simulink library "SUB_ECU_L4_MABX_HW_Interface_PTC_166"  (R2018a)
settings: Solver=VariableStepAuto  StartTime=0.0  StopTime=10.0  RelTol=1e-3
PostLoadFcn:
  | , if any(exist('dsrtsu_mdlpostloadfcn', 'file') == [2, 3, 6]), try dsrtsu_mdlpostloadfcn('Execute', bdroot); catch fprintf('Error in PostLoadFcn (dsrtsu_mdlpostloadfcn) for model "%s":\n %s\n', bdroot, lasterr); end, end,
undefined symbols (not defined in the file or in its folder): CANR_PROPB_REAX_3_13_CHANNEL_APV, CANR_PROPB_REAX_4_13_CHANNEL_APV, CANR_PROPB_XPR_1_50_CHANNEL_APV, ENUM_CAN_RX_T, ENUM_CAN_TX_T, ENUM_REAX_OPERATION_MODE_T, ENUM_SIGNAL_HEALTH_T, ENUM_XBR_CONTROL_MODE_T, ENUM_XBR_EBI_MODE_T, ENUM_XBR_PASS_THROUGH_ACTIVE_T, ENUM_XBR_PRIORITY_T, ENUM_XPR_INHIBIT_PARK_MANUAL_T, ENUM_XPR_INHIBIT_UNPARK_MANUAL_T, ENUM_XPR_PARK_MANUAL_T, ENUM_XPR_UNPARK_MANUAL_T, PROPB_REAX_1_E4_DES_POS_SIG_SRC_APV, PROPB_REAX_1_E4_DESIRED_OPMODE_APV, PROPB_REAX_1_E4_DESIRED_POSITION_APV, ptc_matlab_lib
libraries: PTC_MBDS_LIB x163, rtican x79, simulink x41, EmE_MBD_Blockset x35, rti1401lib_dio_type4 x8, simulink_need_slupdate x7, $bdroot x5, rti1401lib_adc_type4 x3, rtitasklib x1
(part 5 of 25)

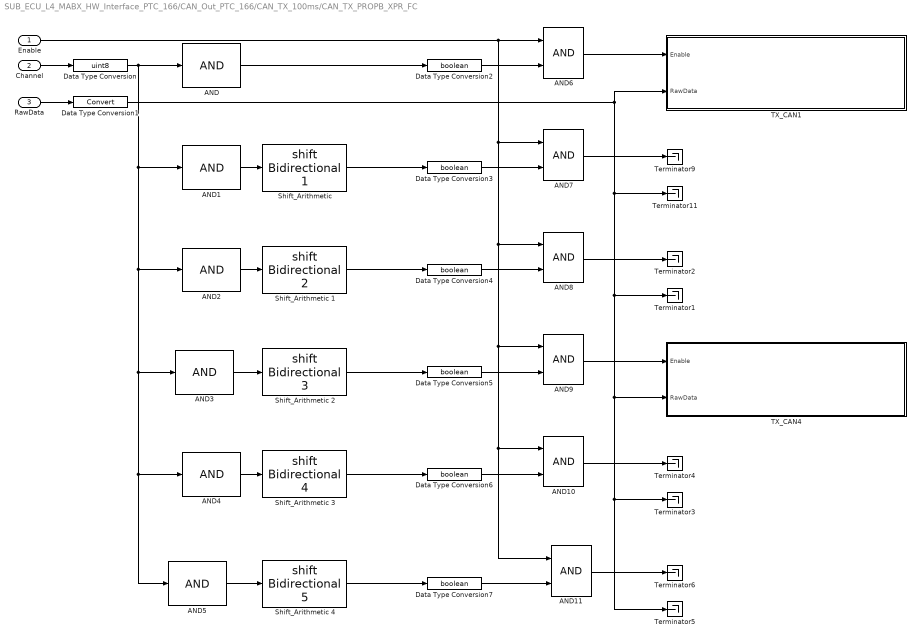
== system SUB_ECU_L4_MABX_HW_Interface_PTC_166/CAN_Out_PTC_166/CAN_TX_100ms/CAN_TX_PROPB_XPR_FC ==
  Enable : Inport
  Channel : Inport  Port=2  OutDataTypeStr=Enum: ENUM_CAN_TX_T
  RawData : Inport  Port=3  OutDataTypeStr=uint8
  AND : PTC_MBDS_LIB/MBDS Standard Library/Basic Operations/Logic and Bit Operations/AND  BitwiseMode=on  Inputs=1  UseBitMask=on  BitMask=bin2dec('00000001')  OutDataTypeStr=Inherit: Inherit via back propagation  PTC_MBDS_BlockVersion=5.41  PTC_BlockType=PTC_MBDS_AND
      settings: AttributesFormatString=bitwise  SourceProductName=PACCAR Technical Center MBDS Library
  AND1 : PTC_MBDS_LIB/MBDS Standard Library/Basic Operations/Logic and Bit Operations/AND  BitwiseMode=on  Inputs=1  UseBitMask=on  BitMask=bin2dec('00000010')  OutDataTypeStr=Inherit: Inherit via back propagation  PTC_MBDS_BlockVersion=5.41  PTC_BlockType=PTC_MBDS_AND
      settings: AttributesFormatString=bitwise  SourceProductName=PACCAR Technical Center MBDS Library
  AND{6..11} (6 alike) : PTC_MBDS_LIB/MBDS Standard Library/Basic Operations/Logic and Bit Operations/AND  BitwiseMode=off  Inputs=2  UseBitMask=off  BitMask='A7'  OutDataTypeStr=Inherit: Inherit via back propagation  PTC_MBDS_BlockVersion=5.41  PTC_BlockType=PTC_MBDS_AND
      settings: SourceProductName=PACCAR Technical Center MBDS Library
  AND2 : PTC_MBDS_LIB/MBDS Standard Library/Basic Operations/Logic and Bit Operations/AND  BitwiseMode=on  Inputs=1  UseBitMask=on  BitMask=bin2dec('00000100')  OutDataTypeStr=Inherit: Inherit via back propagation  PTC_MBDS_BlockVersion=5.41  PTC_BlockType=PTC_MBDS_AND
      settings: AttributesFormatString=bitwise  SourceProductName=PACCAR Technical Center MBDS Library
  AND3 : PTC_MBDS_LIB/MBDS Standard Library/Basic Operations/Logic and Bit Operations/AND  BitwiseMode=on  Inputs=1  UseBitMask=on  BitMask=bin2dec('00001000')  OutDataTypeStr=Inherit: Inherit via back propagation  PTC_MBDS_BlockVersion=5.41  PTC_BlockType=PTC_MBDS_AND
      settings: AttributesFormatString=bitwise  SourceProductName=PACCAR Technical Center MBDS Library
  AND4 : PTC_MBDS_LIB/MBDS Standard Library/Basic Operations/Logic and Bit Operations/AND  BitwiseMode=on  Inputs=1  UseBitMask=on  BitMask=bin2dec('00010000')  OutDataTypeStr=Inherit: Inherit via back propagation  PTC_MBDS_BlockVersion=5.41  PTC_BlockType=PTC_MBDS_AND
      settings: AttributesFormatString=bitwise  SourceProductName=PACCAR Technical Center MBDS Library
  AND5 : PTC_MBDS_LIB/MBDS Standard Library/Basic Operations/Logic and Bit Operations/AND  BitwiseMode=on  Inputs=1  UseBitMask=on  BitMask=bin2dec('00100000')  OutDataTypeStr=Inherit: Inherit via back propagation  PTC_MBDS_BlockVersion=5.41  PTC_BlockType=PTC_MBDS_AND
      settings: AttributesFormatString=bitwise  SourceProductName=PACCAR Technical Center MBDS Library
  Data Type Conversion : DataTypeConversion  OutDataTypeStr=uint8  SaturateOnIntegerOverflow=on
  Data Type Conversion1 : DataTypeConversion  SaturateOnIntegerOverflow=on
  Data Type Conversion{2..7} (6 alike) : DataTypeConversion  OutDataTypeStr=boolean  SaturateOnIntegerOverflow=on
  "Shift_Arithmetic " : ArithShift  BitShiftNumber=1
  Shift_Arithmetic 1 : ArithShift  BitShiftNumber=2
  Shift_Arithmetic 2 : ArithShift  BitShiftNumber=3
  Shift_Arithmetic 3 : ArithShift  BitShiftNumber=4
  Shift_Arithmetic 4 : ArithShift  BitShiftNumber=5
  TX_CAN1 : Subsystem
  TX_CAN4 : Subsystem
  Terminator{1..6,9,11} (8 alike) : Terminator
  wires:
  Shift_Arithmetic 4/1 -> Data Type Conversion7/1
  AND5/1 -> Shift_Arithmetic 4/1
  Shift_Arithmetic 3/1 -> Data Type Conversion6/1
  AND4/1 -> Shift_Arithmetic 3/1
  Shift_Arithmetic 2/1 -> Data Type Conversion5/1
  AND3/1 -> Shift_Arithmetic 2/1
  Shift_Arithmetic 1/1 -> Data Type Conversion4/1
  "Shift_Arithmetic "/1 -> Data Type Conversion3/1
  AND/1 -> Data Type Conversion2/1
  RawData/1 -> Data Type Conversion1/1
  Data Type Conversion/1 -> AND2/1, AND3/1, AND5/1, AND4/1, AND1/1, AND/1
  Channel/1 -> Data Type Conversion/1
  AND2/1 -> Shift_Arithmetic 1/1
  AND1/1 -> "Shift_Arithmetic "/1
  Data Type Conversion1/1 -> TX_CAN1/2(RawData), Terminator11/1, Terminator1/1, TX_CAN4/2(RawData), Terminator5/1, Terminator3/1
  Data Type Conversion2/1 -> AND6/2
  Data Type Conversion3/1 -> AND7/2
  Data Type Conversion4/1 -> AND8/2
  Data Type Conversion5/1 -> AND9/2
  Data Type Conversion6/1 -> AND10/2
  Data Type Conversion7/1 -> AND11/2
  Enable/1 -> AND11/1, AND10/1, AND9/1, AND8/1, AND7/1, AND6/1
  AND11/1 -> Terminator6/1
  AND10/1 -> Terminator4/1
  AND9/1 -> TX_CAN4/1(Enable)
  AND8/1 -> Terminator2/1
  AND7/1 -> Terminator9/1
  AND6/1 -> TX_CAN1/1(Enable)

== system SUB_ECU_L4_MABX_HW_Interface_PTC_166/CAN_Out_PTC_166/CAN_TX_100ms/COGSRapidUpdate ==
  Enable : Inport
  Data : Inport  Port=2
  Data Type Conversion2 : DataTypeConversion  OutDataTypeStr=boolean  SaturateOnIntegerOverflow=on
  TX : Subsystem
  wires:
  Enable/1 -> Data Type Conversion2/1
  Data/1 -> TX/2(Data)
  Data Type Conversion2/1 -> TX/1(Enable)

== system SUB_ECU_L4_MABX_HW_Interface_PTC_166/CAN_Out_PTC_166/CAN_TX_100ms/EBC1_8B ==
  Enable : Inport
  Data : Inport  Port=2
  Data Type Conversion2 : DataTypeConversion  OutDataTypeStr=boolean  SaturateOnIntegerOverflow=on
  TX_EBC1_8B : Subsystem
  wires:
  Data Type Conversion2/1 -> TX_EBC1_8B/1(Enable)
  Data/1 -> TX_EBC1_8B/2(Data)
  Enable/1 -> Data Type Conversion2/1

== system SUB_ECU_L4_MABX_HW_Interface_PTC_166/CAN_Out_PTC_166/CAN_TX_100ms/EffortsValue ==
  Constant : Constant  Value=int16(512)
  EffortsValue : Outport
  wires:
  Constant/1 -> EffortsValue/1

== system SUB_ECU_L4_MABX_HW_Interface_PTC_166/CAN_Out_PTC_166/CAN_TX_100ms/Encode_PropB_REAX_5 ==
  EffortsValue : Inport
  AND : PTC_MBDS_LIB/MBDS Standard Library/Basic Operations/Logic and Bit Operations/AND  BitwiseMode=on  Inputs=1  UseBitMask=on  BitMask='00FF'  OutDataTypeStr=uint8  PTC_MBDS_BlockVersion=5.41  PTC_BlockType=PTC_MBDS_AND
      settings: AttributesFormatString=bitwise  SourceProductName=PACCAR Technical Center MBDS Library
  AND1 : PTC_MBDS_LIB/MBDS Standard Library/Basic Operations/Logic and Bit Operations/AND  BitwiseMode=on  Inputs=1  UseBitMask=on  BitMask='FF00'  OutDataTypeStr=uint16  PTC_MBDS_BlockVersion=5.41  PTC_BlockType=PTC_MBDS_AND
      settings: AttributesFormatString=bitwise  SourceProductName=PACCAR Technical Center MBDS Library
  Constant : Constant  Value=uint8(hex2dec('FF'))
  Data Type Conversion : DataTypeConversion  OutDataTypeStr=int16  SaturateOnIntegerOverflow=on
  Data Type Conversion1 : DataTypeConversion  OutDataTypeStr=uint16  ConvertRealWorld=Stored Integer (SI)
  Data Type Conversion2 : DataTypeConversion  OutDataTypeStr=uint8  SaturateOnIntegerOverflow=on
  Mux : Mux  Inputs=8
  "Shift_Arithmetic " : ArithShift  BitShiftNumber=8
  Data : Outport
  wires:
  Mux/1 -> Data/1
  Constant/1 -> Mux/1, Mux/2, Mux/4, Mux/5, Mux/6, Mux/3
  Data Type Conversion2/1 -> Mux/8
  AND/1 -> Mux/7
  "Shift_Arithmetic "/1 -> Data Type Conversion2/1
  AND1/1 -> "Shift_Arithmetic "/1
  Data Type Conversion1/1 -> AND/1, AND1/1
  Data Type Conversion/1 -> Data Type Conversion1/1
  EffortsValue/1 -> Data Type Conversion/1

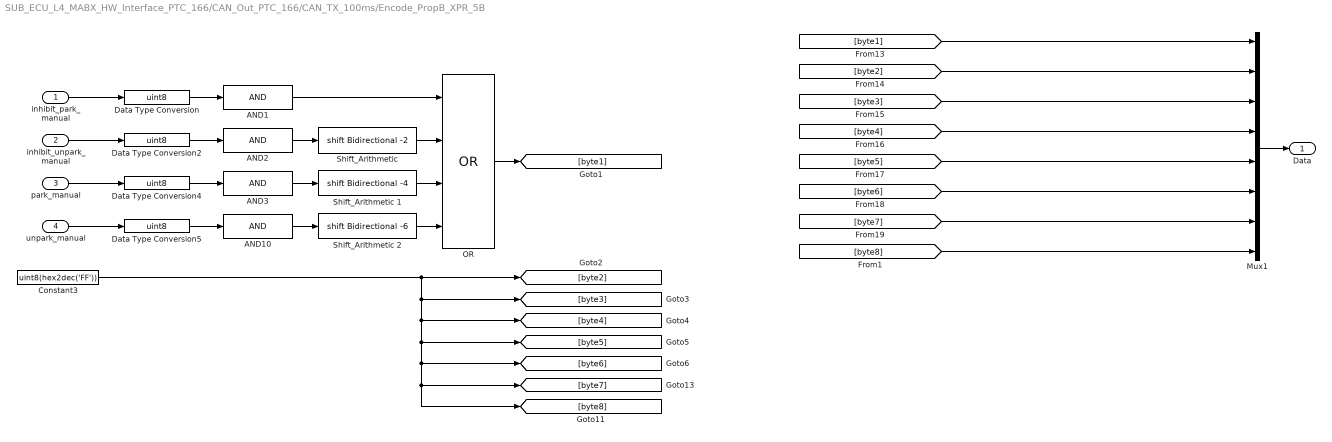
== system SUB_ECU_L4_MABX_HW_Interface_PTC_166/CAN_Out_PTC_166/CAN_TX_100ms/Encode_PropB_XPR_5B ==
  inhibit_park_manual : Inport
  inhibit_unpark_manual : Inport  Port=2
  park_manual : Inport  Port=3
  unpark_manual : Inport  Port=4
  AND{1..3,10} (4 alike) : PTC_MBDS_LIB/MBDS Standard Library/Basic Operations/Logic and Bit Operations/AND  BitwiseMode=on  Inputs=1  UseBitMask=on  BitMask=bin2dec('00000011')  OutDataTypeStr=uint8  PTC_MBDS_BlockVersion=5.41  PTC_BlockType=PTC_MBDS_AND
      settings: AttributesFormatString=bitwise  SourceProductName=PACCAR Technical Center MBDS Library
  Constant3 : Constant  Value=uint8(hex2dec('FF'))
  Data Type Conversion{,2,4..5} (4 alike) : DataTypeConversion  OutMin=0  OutMax=3  OutDataTypeStr=uint8  SaturateOnIntegerOverflow=on
  Mux1 : Mux  Inputs=8
  OR : PTC_MBDS_LIB/MBDS Standard Library/Basic Operations/Logic and Bit Operations/OR  BitwiseMode=on  Inputs=4  UseBitMask=off  BitMask='A7'  OutDataTypeStr=uint8  PTC_MBDS_BlockVersion=5.41  PTC_BlockType=PTC_MBDS_OR
      settings: AttributesFormatString=bitwise  SourceProductName=PACCAR Technical Center MBDS Library
  "Shift_Arithmetic " : ArithShift  BitShiftNumber=-2
  Shift_Arithmetic 1 : ArithShift  BitShiftNumber=-4
  Shift_Arithmetic 2 : ArithShift  BitShiftNumber=-6
  Data : Outport
  wires:
  [byte8] -> Mux1/8
  AND10/1 -> Shift_Arithmetic 2/1
  AND3/1 -> Shift_Arithmetic 1/1
  AND2/1 -> "Shift_Arithmetic "/1
  AND1/1 -> OR/1
  Data Type Conversion5/1 -> AND10/1
  Data Type Conversion4/1 -> AND3/1
  Data Type Conversion2/1 -> AND2/1
  OR/1 -> [byte1]
  Shift_Arithmetic 2/1 -> OR/4
  Shift_Arithmetic 1/1 -> OR/3
  Data Type Conversion/1 -> AND1/1
  "Shift_Arithmetic "/1 -> OR/2
  unpark_manual/1 -> Data Type Conversion5/1
  park_manual/1 -> Data Type Conversion4/1
  inhibit_unpark_manual/1 -> Data Type Conversion2/1
  inhibit_park_manual/1 -> Data Type Conversion/1
  [byte6] -> Mux1/6
  [byte5] -> Mux1/5
  [byte4] -> Mux1/4
  [byte3] -> Mux1/3
  [byte2] -> Mux1/2
  [byte1] -> Mux1/1
  Constant3/1 -> [byte2], [byte3], [byte4], [byte5], [byte6], [byte7], [byte8]
  Mux1/1 -> Data/1
  [byte7] -> Mux1/7

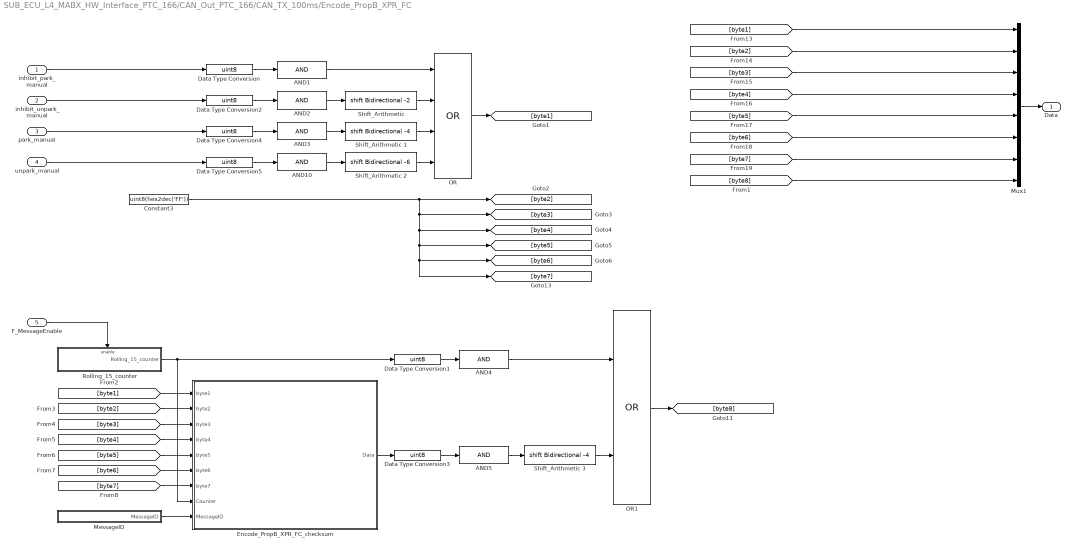
== system SUB_ECU_L4_MABX_HW_Interface_PTC_166/CAN_Out_PTC_166/CAN_TX_100ms/Encode_PropB_XPR_FC ==
  inhibit_park_manual : Inport
  inhibit_unpark_manual : Inport  Port=2
  park_manual : Inport  Port=3
  unpark_manual : Inport  Port=4
  F_MessageEnable : Inport  Port=5
  AND{1..3,10} (4 alike) : PTC_MBDS_LIB/MBDS Standard Library/Basic Operations/Logic and Bit Operations/AND  BitwiseMode=on  Inputs=1  UseBitMask=on  BitMask=bin2dec('00000011')  OutDataTypeStr=uint8  PTC_MBDS_BlockVersion=5.41  PTC_BlockType=PTC_MBDS_AND
      settings: AttributesFormatString=bitwise  SourceProductName=PACCAR Technical Center MBDS Library
  AND4 : PTC_MBDS_LIB/MBDS Standard Library/Basic Operations/Logic and Bit Operations/AND  BitwiseMode=on  Inputs=1  UseBitMask=on  BitMask=bin2dec('00001111')  OutDataTypeStr=uint8  PTC_MBDS_BlockVersion=5.41  PTC_BlockType=PTC_MBDS_AND
      settings: AttributesFormatString=bitwise  SourceProductName=PACCAR Technical Center MBDS Library
  AND5 : PTC_MBDS_LIB/MBDS Standard Library/Basic Operations/Logic and Bit Operations/AND  BitwiseMode=on  Inputs=1  UseBitMask=on  BitMask=bin2dec('00001111')  OutDataTypeStr=uint8  PTC_MBDS_BlockVersion=5.41  PTC_BlockType=PTC_MBDS_AND
      settings: AttributesFormatString=bitwise  SourceProductName=PACCAR Technical Center MBDS Library
  Constant3 : Constant  Value=uint8(hex2dec('FF'))
  Data Type Conversion{,1..5} (6 alike) : DataTypeConversion  OutMin=0  OutMax=3  OutDataTypeStr=uint8  SaturateOnIntegerOverflow=on
  Encode_PropB_XPR_FC_checksum : Subsystem
  MessageID : Subsystem
  Mux1 : Mux  Inputs=8
  OR : PTC_MBDS_LIB/MBDS Standard Library/Basic Operations/Logic and Bit Operations/OR  BitwiseMode=on  Inputs=4  UseBitMask=off  BitMask='A7'  OutDataTypeStr=uint8  PTC_MBDS_BlockVersion=5.41  PTC_BlockType=PTC_MBDS_OR
      settings: AttributesFormatString=bitwise  SourceProductName=PACCAR Technical Center MBDS Library
  OR1 : PTC_MBDS_LIB/MBDS Standard Library/Basic Operations/Logic and Bit Operations/OR  BitwiseMode=on  Inputs=2  UseBitMask=off  BitMask='A7'  OutDataTypeStr=uint8  PTC_MBDS_BlockVersion=5.41  PTC_BlockType=PTC_MBDS_OR
      settings: AttributesFormatString=bitwise  SourceProductName=PACCAR Technical Center MBDS Library
  Rolling_15_counter : Subsystem
  "Shift_Arithmetic " : ArithShift  BitShiftNumber=-2
  Shift_Arithmetic 1 : ArithShift  BitShiftNumber=-4
  Shift_Arithmetic 2 : ArithShift  BitShiftNumber=-6
  Shift_Arithmetic 3 : ArithShift  BitShiftNumber=-4
  Data : Outport
  wires:
  [byte8] -> Mux1/8
  AND10/1 -> Shift_Arithmetic 2/1
  AND3/1 -> Shift_Arithmetic 1/1
  AND2/1 -> "Shift_Arithmetic "/1
  AND1/1 -> OR/1
  Data Type Conversion5/1 -> AND10/1
  Data Type Conversion4/1 -> AND3/1
  Data Type Conversion2/1 -> AND2/1
  OR/1 -> [byte1]
  Shift_Arithmetic 2/1 -> OR/4
  Shift_Arithmetic 1/1 -> OR/3
  Data Type Conversion/1 -> AND1/1
  "Shift_Arithmetic "/1 -> OR/2
  unpark_manual/1 -> Data Type Conversion5/1
  park_manual/1 -> Data Type Conversion4/1
  inhibit_unpark_manual/1 -> Data Type Conversion2/1
  inhibit_park_manual/1 -> Data Type Conversion/1
  [byte6] -> Mux1/6
  [byte5] -> Mux1/5
  [byte4] -> Mux1/4
  [byte3] -> Mux1/3
  [byte2] -> Mux1/2
  [byte1] -> Mux1/1
  Constant3/1 -> [byte2], [byte3], [byte4], [byte5], [byte6], [byte7]
  Mux1/1 -> Data/1
  [byte7] -> Mux1/7
  Rolling_15_counter/1(Rolling_15_counter) -> Data Type Conversion1/1, Encode_PropB_XPR_FC_checksum/8(Counter)
  MessageID/1(MessageID) -> Encode_PropB_XPR_FC_checksum/9(MessageID)
  Data Type Conversion1/1 -> AND4/1
  Data Type Conversion3/1 -> AND5/1
  Encode_PropB_XPR_FC_checksum/1(Data) -> Data Type Conversion3/1
  AND5/1 -> Shift_Arithmetic 3/1
  AND4/1 -> OR1/1
  Shift_Arithmetic 3/1 -> OR1/2
  OR1/1 -> [byte8]
  [byte7] -> Encode_PropB_XPR_FC_checksum/7(byte7)
  [byte6] -> Encode_PropB_XPR_FC_checksum/6(byte6)
  [byte5] -> Encode_PropB_XPR_FC_checksum/5(byte5)
  [byte4] -> Encode_PropB_XPR_FC_checksum/4(byte4)
  [byte3] -> Encode_PropB_XPR_FC_checksum/3(byte3)
  [byte2] -> Encode_PropB_XPR_FC_checksum/2(byte2)
  [byte1] -> Encode_PropB_XPR_FC_checksum/1(byte1)
  F_MessageEnable/1 -> Rolling_15_counter/Enable

== system SUB_ECU_L4_MABX_HW_Interface_PTC_166/CAN_Out_PTC_166/CAN_TX_100ms/POSRapidUpdate ==
  Enable : Inport
  Data : Inport  Port=2
  Data Type Conversion2 : DataTypeConversion  OutDataTypeStr=boolean  SaturateOnIntegerOverflow=on
  TX : Subsystem
  wires:
  Data Type Conversion2/1 -> TX/1(Enable)
  Data/1 -> TX/2(Data)
  Enable/1 -> Data Type Conversion2/1

== system SUB_ECU_L4_MABX_HW_Interface_PTC_166/CAN_Out_PTC_166/CAN_TX_10ms/CAN_TX_ACCS_E4 ==
  Channel : Inport  OutDataTypeStr=Enum: ENUM_CAN_TX_T
  Data : Inport  Port=2
  AND : PTC_MBDS_LIB/MBDS Standard Library/Basic Operations/Logic and Bit Operations/AND  BitwiseMode=on  Inputs=1  UseBitMask=on  BitMask=bin2dec('00000001')  OutDataTypeStr=Inherit: Inherit via back propagation  PTC_MBDS_BlockVersion=5.41  PTC_BlockType=PTC_MBDS_AND
      settings: AttributesFormatString=bitwise  SourceProductName=PACCAR Technical Center MBDS Library
  AND1 : PTC_MBDS_LIB/MBDS Standard Library/Basic Operations/Logic and Bit Operations/AND  BitwiseMode=on  Inputs=1  UseBitMask=on  BitMask=bin2dec('00000010')  OutDataTypeStr=Inherit: Inherit via back propagation  PTC_MBDS_BlockVersion=5.41  PTC_BlockType=PTC_MBDS_AND
      settings: AttributesFormatString=bitwise  SourceProductName=PACCAR Technical Center MBDS Library
  AND2 : PTC_MBDS_LIB/MBDS Standard Library/Basic Operations/Logic and Bit Operations/AND  BitwiseMode=on  Inputs=1  UseBitMask=on  BitMask=bin2dec('00000100')  OutDataTypeStr=Inherit: Inherit via back propagation  PTC_MBDS_BlockVersion=5.41  PTC_BlockType=PTC_MBDS_AND
      settings: AttributesFormatString=bitwise  SourceProductName=PACCAR Technical Center MBDS Library
  AND3 : PTC_MBDS_LIB/MBDS Standard Library/Basic Operations/Logic and Bit Operations/AND  BitwiseMode=on  Inputs=1  UseBitMask=on  BitMask=bin2dec('00001000')  OutDataTypeStr=Inherit: Inherit via back propagation  PTC_MBDS_BlockVersion=5.41  PTC_BlockType=PTC_MBDS_AND
      settings: AttributesFormatString=bitwise  SourceProductName=PACCAR Technical Center MBDS Library
  AND4 : PTC_MBDS_LIB/MBDS Standard Library/Basic Operations/Logic and Bit Operations/AND  BitwiseMode=on  Inputs=1  UseBitMask=on  BitMask=bin2dec('00010000')  OutDataTypeStr=Inherit: Inherit via back propagation  PTC_MBDS_BlockVersion=5.41  PTC_BlockType=PTC_MBDS_AND
      settings: AttributesFormatString=bitwise  SourceProductName=PACCAR Technical Center MBDS Library
  AND5 : PTC_MBDS_LIB/MBDS Standard Library/Basic Operations/Logic and Bit Operations/AND  BitwiseMode=on  Inputs=1  UseBitMask=on  BitMask=bin2dec('00100000')  OutDataTypeStr=Inherit: Inherit via back propagation  PTC_MBDS_BlockVersion=5.41  PTC_BlockType=PTC_MBDS_AND
      settings: AttributesFormatString=bitwise  SourceProductName=PACCAR Technical Center MBDS Library
  Data Type Conversion : DataTypeConversion  OutDataTypeStr=uint8  SaturateOnIntegerOverflow=on
  Data Type Conversion{2..7} (6 alike) : DataTypeConversion  OutDataTypeStr=boolean  SaturateOnIntegerOverflow=on
  "Shift_Arithmetic " : ArithShift  BitShiftNumber=1
  Shift_Arithmetic 1 : ArithShift  BitShiftNumber=2
  Shift_Arithmetic 2 : ArithShift  BitShiftNumber=3
  Shift_Arithmetic 3 : ArithShift  BitShiftNumber=4
  Shift_Arithmetic 4 : ArithShift  BitShiftNumber=5
  TX_CAN4 : Subsystem
  Terminator{,1..9} (10 alike) : Terminator
  wires:
  AND1/1 -> "Shift_Arithmetic "/1
  AND2/1 -> Shift_Arithmetic 1/1
  Channel/1 -> Data Type Conversion/1
  Data Type Conversion/1 -> AND/1, AND1/1, AND5/1, AND4/1, AND3/1, AND2/1
  AND/1 -> Data Type Conversion2/1
  "Shift_Arithmetic "/1 -> Data Type Conversion3/1
  Shift_Arithmetic 1/1 -> Data Type Conversion4/1
  AND3/1 -> Shift_Arithmetic 2/1
  Shift_Arithmetic 2/1 -> Data Type Conversion5/1
  AND4/1 -> Shift_Arithmetic 3/1
  Shift_Arithmetic 3/1 -> Data Type Conversion6/1
  AND5/1 -> Shift_Arithmetic 4/1
  Shift_Arithmetic 4/1 -> Data Type Conversion7/1
  Data/1 -> Terminator9/1, Terminator5/1, TX_CAN4/2(Data), Terminator7/1, Terminator3/1, Terminator1/1
  Data Type Conversion2/1 -> Terminator/1
  Data Type Conversion3/1 -> Terminator2/1
  Data Type Conversion4/1 -> Terminator6/1
  Data Type Conversion5/1 -> TX_CAN4/1(Enable)
  Data Type Conversion6/1 -> Terminator4/1
  Data Type Conversion7/1 -> Terminator8/1

== system SUB_ECU_L4_MABX_HW_Interface_PTC_166/CAN_Out_PTC_166/CAN_TX_10ms/CAN_TX_EEC1_00 ==
  Channel : Inport  OutDataTypeStr=Enum: ENUM_CAN_TX_T
  Data : Inport  Port=2
  AND : PTC_MBDS_LIB/MBDS Standard Library/Basic Operations/Logic and Bit Operations/AND  BitwiseMode=on  Inputs=1  UseBitMask=on  BitMask=bin2dec('00000001')  OutDataTypeStr=Inherit: Inherit via back propagation  PTC_MBDS_BlockVersion=5.41  PTC_BlockType=PTC_MBDS_AND
      settings: AttributesFormatString=bitwise  SourceProductName=PACCAR Technical Center MBDS Library
  AND1 : PTC_MBDS_LIB/MBDS Standard Library/Basic Operations/Logic and Bit Operations/AND  BitwiseMode=on  Inputs=1  UseBitMask=on  BitMask=bin2dec('00000010')  OutDataTypeStr=Inherit: Inherit via back propagation  PTC_MBDS_BlockVersion=5.41  PTC_BlockType=PTC_MBDS_AND
      settings: AttributesFormatString=bitwise  SourceProductName=PACCAR Technical Center MBDS Library
  AND2 : PTC_MBDS_LIB/MBDS Standard Library/Basic Operations/Logic and Bit Operations/AND  BitwiseMode=on  Inputs=1  UseBitMask=on  BitMask=bin2dec('00000100')  OutDataTypeStr=Inherit: Inherit via back propagation  PTC_MBDS_BlockVersion=5.41  PTC_BlockType=PTC_MBDS_AND
      settings: AttributesFormatString=bitwise  SourceProductName=PACCAR Technical Center MBDS Library
  AND3 : PTC_MBDS_LIB/MBDS Standard Library/Basic Operations/Logic and Bit Operations/AND  BitwiseMode=on  Inputs=1  UseBitMask=on  BitMask=bin2dec('00001000')  OutDataTypeStr=Inherit: Inherit via back propagation  PTC_MBDS_BlockVersion=5.41  PTC_BlockType=PTC_MBDS_AND
      settings: AttributesFormatString=bitwise  SourceProductName=PACCAR Technical Center MBDS Library
  AND4 : PTC_MBDS_LIB/MBDS Standard Library/Basic Operations/Logic and Bit Operations/AND  BitwiseMode=on  Inputs=1  UseBitMask=on  BitMask=bin2dec('00010000')  OutDataTypeStr=Inherit: Inherit via back propagation  PTC_MBDS_BlockVersion=5.41  PTC_BlockType=PTC_MBDS_AND
      settings: AttributesFormatString=bitwise  SourceProductName=PACCAR Technical Center MBDS Library
  AND5 : PTC_MBDS_LIB/MBDS Standard Library/Basic Operations/Logic and Bit Operations/AND  BitwiseMode=on  Inputs=1  UseBitMask=on  BitMask=bin2dec('00100000')  OutDataTypeStr=Inherit: Inherit via back propagation  PTC_MBDS_BlockVersion=5.41  PTC_BlockType=PTC_MBDS_AND
      settings: AttributesFormatString=bitwise  SourceProductName=PACCAR Technical Center MBDS Library
  Data Type Conversion : DataTypeConversion  OutDataTypeStr=uint8  SaturateOnIntegerOverflow=on
  Data Type Conversion{2..7} (6 alike) : DataTypeConversion  OutDataTypeStr=boolean  SaturateOnIntegerOverflow=on
  "Shift_Arithmetic " : ArithShift  BitShiftNumber=1
  Shift_Arithmetic 1 : ArithShift  BitShiftNumber=2
  Shift_Arithmetic 2 : ArithShift  BitShiftNumber=3
  Shift_Arithmetic 3 : ArithShift  BitShiftNumber=4
  Shift_Arithmetic 4 : ArithShift  BitShiftNumber=5
  TX_CAN4 : Subsystem
  TX_CAN5 : Subsystem
  Terminator{,1..3,6..9} (8 alike) : Terminator
  wires:
  Data Type Conversion7/1 -> Terminator8/1
  Data Type Conversion6/1 -> TX_CAN5/1(Enable)
  Data Type Conversion5/1 -> TX_CAN4/1(Enable)
  Data Type Conversion4/1 -> Terminator6/1
  Data Type Conversion3/1 -> Terminator2/1
  Data Type Conversion2/1 -> Terminator/1
  Data/1 -> Terminator1/1, Terminator3/1, Terminator7/1, TX_CAN4/2(Data), TX_CAN5/2(Data), Terminator9/1
  Shift_Arithmetic 4/1 -> Data Type Conversion7/1
  AND5/1 -> Shift_Arithmetic 4/1
  Shift_Arithmetic 3/1 -> Data Type Conversion6/1
  AND4/1 -> Shift_Arithmetic 3/1
  Shift_Arithmetic 2/1 -> Data Type Conversion5/1
  AND3/1 -> Shift_Arithmetic 2/1
  Shift_Arithmetic 1/1 -> Data Type Conversion4/1
  "Shift_Arithmetic "/1 -> Data Type Conversion3/1
  AND/1 -> Data Type Conversion2/1
  Data Type Conversion/1 -> AND2/1, AND3/1, AND4/1, AND5/1, AND1/1, AND/1
  Channel/1 -> Data Type Conversion/1
  AND2/1 -> Shift_Arithmetic 1/1
  AND1/1 -> "Shift_Arithmetic "/1

== system SUB_ECU_L4_MABX_HW_Interface_PTC_166/CAN_Out_PTC_166/CAN_TX_10ms/CAN_TX_PROPB_REAX_1_E4 ==
  enable : Inport
  RawData : Inport  Port=2  OutDataTypeStr=uint8
  Data Type Conversion1 : DataTypeConversion  SaturateOnIntegerOverflow=on
  Ground : Ground
  Ground1 : Ground
  TX_CAN4 : Subsystem
  TX_CAN5 : Subsystem
  Terminator : Terminator
  wires:
  Data Type Conversion1/1 -> TX_CAN5/2(RawData), TX_CAN4/2(RawData)
  RawData/1 -> Data Type Conversion1/1
  enable/1 -> Terminator/1
  Ground/1 -> TX_CAN4/1(Enable)  "EnablePropB_ReAX_CAN4"
  Ground1/1 -> TX_CAN5/1(Enable)  "EnablePropB_ReAX_CAN5"

== system SUB_ECU_L4_MABX_HW_Interface_PTC_166/CAN_Out_PTC_166/CAN_TX_10ms/CAN_TX_VDC2_0B ==
  Channel : Inport  OutDataTypeStr=Enum: ENUM_CAN_TX_T
  Data : Inport  Port=2
  AND : PTC_MBDS_LIB/MBDS Standard Library/Basic Operations/Logic and Bit Operations/AND  BitwiseMode=on  Inputs=1  UseBitMask=on  BitMask=bin2dec('00000001')  OutDataTypeStr=Inherit: Inherit via back propagation  PTC_MBDS_BlockVersion=5.41  PTC_BlockType=PTC_MBDS_AND
      settings: AttributesFormatString=bitwise  SourceProductName=PACCAR Technical Center MBDS Library
  AND1 : PTC_MBDS_LIB/MBDS Standard Library/Basic Operations/Logic and Bit Operations/AND  BitwiseMode=on  Inputs=1  UseBitMask=on  BitMask=bin2dec('00000010')  OutDataTypeStr=Inherit: Inherit via back propagation  PTC_MBDS_BlockVersion=5.41  PTC_BlockType=PTC_MBDS_AND
      settings: AttributesFormatString=bitwise  SourceProductName=PACCAR Technical Center MBDS Library
  AND2 : PTC_MBDS_LIB/MBDS Standard Library/Basic Operations/Logic and Bit Operations/AND  BitwiseMode=on  Inputs=1  UseBitMask=on  BitMask=bin2dec('00000100')  OutDataTypeStr=Inherit: Inherit via back propagation  PTC_MBDS_BlockVersion=5.41  PTC_BlockType=PTC_MBDS_AND
      settings: AttributesFormatString=bitwise  SourceProductName=PACCAR Technical Center MBDS Library
  AND3 : PTC_MBDS_LIB/MBDS Standard Library/Basic Operations/Logic and Bit Operations/AND  BitwiseMode=on  Inputs=1  UseBitMask=on  BitMask=bin2dec('00001000')  OutDataTypeStr=Inherit: Inherit via back propagation  PTC_MBDS_BlockVersion=5.41  PTC_BlockType=PTC_MBDS_AND
      settings: AttributesFormatString=bitwise  SourceProductName=PACCAR Technical Center MBDS Library
  AND4 : PTC_MBDS_LIB/MBDS Standard Library/Basic Operations/Logic and Bit Operations/AND  BitwiseMode=on  Inputs=1  UseBitMask=on  BitMask=bin2dec('00010000')  OutDataTypeStr=Inherit: Inherit via back propagation  PTC_MBDS_BlockVersion=5.41  PTC_BlockType=PTC_MBDS_AND
      settings: AttributesFormatString=bitwise  SourceProductName=PACCAR Technical Center MBDS Library
  AND5 : PTC_MBDS_LIB/MBDS Standard Library/Basic Operations/Logic and Bit Operations/AND  BitwiseMode=on  Inputs=1  UseBitMask=on  BitMask=bin2dec('00100000')  OutDataTypeStr=Inherit: Inherit via back propagation  PTC_MBDS_BlockVersion=5.41  PTC_BlockType=PTC_MBDS_AND
      settings: AttributesFormatString=bitwise  SourceProductName=PACCAR Technical Center MBDS Library
  Data Type Conversion : DataTypeConversion  OutDataTypeStr=uint8  SaturateOnIntegerOverflow=on
  Data Type Conversion{1,3..7} (6 alike) : DataTypeConversion  OutDataTypeStr=boolean  SaturateOnIntegerOverflow=on
  "Shift_Arithmetic " : ArithShift  BitShiftNumber=1
  Shift_Arithmetic 1 : ArithShift  BitShiftNumber=2
  Shift_Arithmetic 2 : ArithShift  BitShiftNumber=3
  Shift_Arithmetic 3 : ArithShift  BitShiftNumber=4
  Shift_Arithmetic 4 : ArithShift  BitShiftNumber=5
  TX_CAN5 : Subsystem
  Terminator{,1..9} (10 alike) : Terminator
  wires:
  Data Type Conversion7/1 -> Terminator8/1
  Data Type Conversion6/1 -> TX_CAN5/1(Enable)
  Data Type Conversion5/1 -> Terminator6/1
  Data Type Conversion4/1 -> Terminator4/1
  Data Type Conversion3/1 -> Terminator2/1
  Data Type Conversion1/1 -> Terminator/1
  Data/1 -> Terminator1/1, Terminator3/1, Terminator5/1, Terminator7/1, Terminator9/1, TX_CAN5/2(Data)
  Shift_Arithmetic 4/1 -> Data Type Conversion7/1
  AND5/1 -> Shift_Arithmetic 4/1
  Shift_Arithmetic 3/1 -> Data Type Conversion6/1
  AND4/1 -> Shift_Arithmetic 3/1
  Shift_Arithmetic 2/1 -> Data Type Conversion5/1
  AND3/1 -> Shift_Arithmetic 2/1
  Shift_Arithmetic 1/1 -> Data Type Conversion4/1
  "Shift_Arithmetic "/1 -> Data Type Conversion3/1
  AND/1 -> Data Type Conversion1/1
  Data Type Conversion/1 -> AND2/1, AND3/1, AND4/1, AND5/1, AND1/1, AND/1
  Channel/1 -> Data Type Conversion/1
  AND2/1 -> Shift_Arithmetic 1/1
  AND1/1 -> "Shift_Arithmetic "/1

== system SUB_ECU_L4_MABX_HW_Interface_PTC_166/CAN_Out_PTC_166/CAN_TX_10ms/Encode_PROPB_REAX_1 ==
  In1 : Inport
  Bus Selector : BusSelector  OutputSignals=10msTask.SteeringControl.DesSteeringAngle
  Bus Selector1 : BusSelector  OutputSignals=INPUTS.DIO_Bus.OperatorEnableSwitch
  CAN_ID_PropB_REAX_1_E4 : Subsystem
  Data Type Conversion : DataTypeConversion  OutDataTypeStr=uint8
  Encode_PROPB_REAX_1 : Subsystem
  PropB_REAX_1_E4_CommandFromExternalController : Subsystem
  PropB_REAX_1_E4_DesiredOperatingMode : Subsystem
  PropB_REAX_1_E4_MessageCounter : Subsystem
  Out1 : Outport
  wires:
  Data Type Conversion/1 -> PropB_REAX_1_E4_CommandFromExternalController/2(operatorEnable), PropB_REAX_1_E4_DesiredOperatingMode/1(OperatorEnable)
  Bus Selector/1 -> PropB_REAX_1_E4_CommandFromExternalController/1(DesiredSteeringAngle)  "<DesSteeringAngle>"
  Bus Selector1/1 -> Data Type Conversion/1  "<OperatorEnableSwitch>"
  CAN_ID_PropB_REAX_1_E4/1(MessageID) -> Encode_PROPB_REAX_1/1(MessageID)
  PropB_REAX_1_E4_DesiredOperatingMode/1(DesiredOperatingMode) -> Encode_PROPB_REAX_1/2(DesiredOperatingMode)
  Encode_PROPB_REAX_1/1(Data) -> Out1/1
  PropB_REAX_1_E4_MessageCounter/1(MessageCounter) -> Encode_PROPB_REAX_1/4(MessageCounter)
  PropB_REAX_1_E4_CommandFromExternalController/1(CommandFromExternalController) -> Encode_PROPB_REAX_1/3(CommandFromExternalController)
  In1/1 -> Bus Selector1/1, Bus Selector/1

== system SUB_ECU_L4_MABX_HW_Interface_PTC_166/CAN_Out_PTC_166/CAN_TX_20ms/CAN_TX_PROPB_XBR_B3 ==
  Channel : Inport
  Data : Inport  Port=2
  OperatorEnable : Inport  Port=3
  AND : PTC_MBDS_LIB/MBDS Standard Library/Basic Operations/Logic and Bit Operations/AND  BitwiseMode=on  Inputs=1  UseBitMask=on  BitMask=bin2dec('00000001')  OutDataTypeStr=Inherit: Inherit via back propagation  PTC_MBDS_BlockVersion=5.41  PTC_BlockType=PTC_MBDS_AND
      settings: AttributesFormatString=bitwise  SourceProductName=PACCAR Technical Center MBDS Library
  Bus Selector2 : BusSelector  OutputSignals=XBRPassThroughActive
  Compare To Constant : simulink/Logic and Bit Operations/Compare To Constant  relop===  const=ENUM_XBR_PASS_THROUGH_ACTIVE_T.ACTIVE  OutDataTypeStr=boolean
  Data Type Conversion : DataTypeConversion  OutDataTypeStr=uint8  SaturateOnIntegerOverflow=on
  Data Type Conversion2 : DataTypeConversion  OutDataTypeStr=boolean  SaturateOnIntegerOverflow=on
  Logical Operator : Logic  AllPortsSameDT=off  OutDataTypeStr=boolean
  Logical Operator1 : Logic  Operator=OR  AllPortsSameDT=off  OutDataTypeStr=boolean
  Logical Operator7 : Logic  AllPortsSameDT=off  OutDataTypeStr=boolean
  Logical Operator8 : Logic  Operator=NOT  AllPortsSameDT=off  OutDataTypeStr=boolean
  TX_CAN1 : Subsystem
  Terminator : Terminator
  Unit_Delay : UnitDelay  InitialCondition=false  SampleTime=-1
      settings: AttributesFormatString=IC: %<vinit>
  wires:
  Compare To Constant/1 -> Terminator/1
  OperatorEnable/1 -> Unit_Delay/1, Logical Operator8/1, Logical Operator1/2
  Unit_Delay/1 -> Logical Operator7/1
  Logical Operator8/1 -> Logical Operator7/2
  Logical Operator/1 -> TX_CAN1/1(Enable)
  Logical Operator1/1 -> Logical Operator/1
  Logical Operator7/1 -> Logical Operator1/1
  Data Type Conversion2/1 -> Logical Operator/2
  Data/1 -> Bus Selector2/1, TX_CAN1/2(Data)
  Channel/1 -> Data Type Conversion/1
  Data Type Conversion/1 -> AND/1
  AND/1 -> Data Type Conversion2/1
  Bus Selector2/1 -> Compare To Constant/1  "<XBRPassThroughActive>"

== system SUB_ECU_L4_MABX_HW_Interface_PTC_166/CAN_Out_PTC_166/CAN_TX_20ms/CAN_TX_PropB_2C2_XPR_65 ==
  Enable : Inport
  RawData : Inport  Port=2  OutDataTypeStr=uint8
  Data Type Conversion1 : DataTypeConversion  SaturateOnIntegerOverflow=on
  TX_CAN4 : Subsystem
  TX_CAN5 : Subsystem
  wires:
  Enable/1 -> TX_CAN4/1(Enable), TX_CAN5/1(Enable)
  Data Type Conversion1/1 -> TX_CAN4/2(RawData), TX_CAN5/2(RawData)
  RawData/1 -> Data Type Conversion1/1

== system SUB_ECU_L4_MABX_HW_Interface_PTC_166/CAN_Out_PTC_166/CAN_TX_20ms/CAN_TX_STD_ODOMETRY ==
  Channel : Inport
  Data : Inport  Port=2
  AND : PTC_MBDS_LIB/MBDS Standard Library/Basic Operations/Logic and Bit Operations/AND  BitwiseMode=on  Inputs=1  UseBitMask=on  BitMask=bin2dec('00000001')  OutDataTypeStr=Inherit: Inherit via back propagation  PTC_MBDS_BlockVersion=5.41  PTC_BlockType=PTC_MBDS_AND
      settings: AttributesFormatString=bitwise  SourceProductName=PACCAR Technical Center MBDS Library
  AND1 : PTC_MBDS_LIB/MBDS Standard Library/Basic Operations/Logic and Bit Operations/AND  BitwiseMode=on  Inputs=1  UseBitMask=on  BitMask=bin2dec('00000010')  OutDataTypeStr=Inherit: Inherit via back propagation  PTC_MBDS_BlockVersion=5.41  PTC_BlockType=PTC_MBDS_AND
      settings: AttributesFormatString=bitwise  SourceProductName=PACCAR Technical Center MBDS Library
  AND2 : PTC_MBDS_LIB/MBDS Standard Library/Basic Operations/Logic and Bit Operations/AND  BitwiseMode=on  Inputs=1  UseBitMask=on  BitMask=bin2dec('00000100')  OutDataTypeStr=Inherit: Inherit via back propagation  PTC_MBDS_BlockVersion=5.41  PTC_BlockType=PTC_MBDS_AND
      settings: AttributesFormatString=bitwise  SourceProductName=PACCAR Technical Center MBDS Library
  AND3 : PTC_MBDS_LIB/MBDS Standard Library/Basic Operations/Logic and Bit Operations/AND  BitwiseMode=on  Inputs=1  UseBitMask=on  BitMask=bin2dec('00001000')  OutDataTypeStr=Inherit: Inherit via back propagation  PTC_MBDS_BlockVersion=5.41  PTC_BlockType=PTC_MBDS_AND
      settings: AttributesFormatString=bitwise  SourceProductName=PACCAR Technical Center MBDS Library
  AND4 : PTC_MBDS_LIB/MBDS Standard Library/Basic Operations/Logic and Bit Operations/AND  BitwiseMode=on  Inputs=1  UseBitMask=on  BitMask=bin2dec('00010000')  OutDataTypeStr=Inherit: Inherit via back propagation  PTC_MBDS_BlockVersion=5.41  PTC_BlockType=PTC_MBDS_AND
      settings: AttributesFormatString=bitwise  SourceProductName=PACCAR Technical Center MBDS Library
  AND5 : PTC_MBDS_LIB/MBDS Standard Library/Basic Operations/Logic and Bit Operations/AND  BitwiseMode=on  Inputs=1  UseBitMask=on  BitMask=bin2dec('00100000')  OutDataTypeStr=Inherit: Inherit via back propagation  PTC_MBDS_BlockVersion=5.41  PTC_BlockType=PTC_MBDS_AND
      settings: AttributesFormatString=bitwise  SourceProductName=PACCAR Technical Center MBDS Library
  Data Type Conversion : DataTypeConversion  OutDataTypeStr=uint8  SaturateOnIntegerOverflow=on
  Data Type Conversion{2..7} (6 alike) : DataTypeConversion  OutDataTypeStr=boolean  SaturateOnIntegerOverflow=on
  "Shift_Arithmetic " : ArithShift  BitShiftNumber=1
  Shift_Arithmetic 1 : ArithShift  BitShiftNumber=2
  Shift_Arithmetic 2 : ArithShift  BitShiftNumber=3
  Shift_Arithmetic 3 : ArithShift  BitShiftNumber=4
  Shift_Arithmetic 4 : ArithShift  BitShiftNumber=5
  TX_CAN6 : Subsystem
  Terminator{,1..9} (10 alike) : Terminator
  wires:
  Data Type Conversion7/1 -> TX_CAN6/1(Enable)
  Data Type Conversion6/1 -> Terminator5/1
  Data Type Conversion5/1 -> Terminator6/1
  Data Type Conversion4/1 -> Terminator7/1
  Data Type Conversion3/1 -> Terminator8/1
  Data Type Conversion2/1 -> Terminator9/1
  Data/1 -> Terminator4/1, Terminator3/1, Terminator2/1, Terminator1/1, Terminator/1, TX_CAN6/2(Data)
  AND1/1 -> "Shift_Arithmetic "/1
  AND2/1 -> Shift_Arithmetic 1/1
  Channel/1 -> Data Type Conversion/1
  Data Type Conversion/1 -> AND/1, AND1/1, AND4/1, AND5/1, AND3/1, AND2/1
  AND/1 -> Data Type Conversion2/1
  "Shift_Arithmetic "/1 -> Data Type Conversion3/1
  Shift_Arithmetic 1/1 -> Data Type Conversion4/1
  AND3/1 -> Shift_Arithmetic 2/1
  Shift_Arithmetic 2/1 -> Data Type Conversion5/1
  AND4/1 -> Shift_Arithmetic 3/1
  Shift_Arithmetic 3/1 -> Data Type Conversion6/1
  AND5/1 -> Shift_Arithmetic 4/1
  Shift_Arithmetic 4/1 -> Data Type Conversion7/1

== system SUB_ECU_L4_MABX_HW_Interface_PTC_166/CAN_Out_PTC_166/CAN_TX_20ms/Encode_PropB_2C2_XPR ==
  In : Inport
  2C2_OR_VALUE_APV : Constant  Value=0
  BrkControlMode_Active : Constant  Value=2
  BrkControlPriority : Constant  Value=3
  BrkControl_RearAxlePressureProportioning : Constant  Value=0
  Bus Selector : BusSelector  OutputSignals=10msTask.BrakeCtrl.BrakingPID_Y
  CAN_ID_PropB_2C2_XPR_65 : Subsystem
  CPV : EmE_MBD_Blockset/Sources/CPV  conval=true
      settings: SourceProductName=PACCAR EmE MBD Blockset
  Encode_PropB_2C2_XPR : Subsystem
  F_2C2_OR_APV : Constant  Value=false
  Gain : Gain  Gain=100
  If_Then_Else1 : EmE_MBD_Blockset/Signal Routing/If_Then_Else
      settings: SourceProductName=PACCAR EmE MBD Blockset
  PropB_2C2_XPR_MessageCounter : Subsystem
  Saturation : Saturate  UpperLimit=1  LowerLimit=0
      settings: AttributesFormatString=|
      | min: %<LowerLimit>
      | max: %<UpperLimit>
  F_2C2_Enable : Outport
  Out : Outport  Port=2
  wires:
  BrkControl_RearAxlePressureProportioning/1 -> Encode_PropB_2C2_XPR/5(Rear_axle_pressure_reduction_demand)
  BrkControlPriority/1 -> Encode_PropB_2C2_XPR/4(Priority)
  BrkControlMode_Active/1 -> Encode_PropB_2C2_XPR/3(Control_mode)
  Gain/1 -> Encode_PropB_2C2_XPR/2(External_pressure_demand)
  Bus Selector/1 -> If_Then_Else1/3  "<BrakingPID_Y>"
  In/1 -> Bus Selector/1
  CAN_ID_PropB_2C2_XPR_65/1(MessageID) -> Encode_PropB_2C2_XPR/1(MessageID)
  Encode_PropB_2C2_XPR/1(Data) -> Out/1
  PropB_2C2_XPR_MessageCounter/1(MessageCounter) -> Encode_PropB_2C2_XPR/6(MessageCounter)
  F_2C2_OR_APV/1 -> If_Then_Else1/1
  2C2_OR_VALUE_APV/1 -> Saturation/1
  If_Then_Else1/1 -> Gain/1
  Saturation/1 -> If_Then_Else1/2
  CPV/1 -> F_2C2_Enable/1

== system SUB_ECU_L4_MABX_HW_Interface_PTC_166/CAN_Out_PTC_166/CAN_TX_20ms/Encode_PropB_XBR_B3 ==
  note: This might cause a limit cycle, why switch pass through mode based on braking error
  In : Inport
  Bus Creator1 : BusCreator  Inputs=7
  Bus Creator2 : BusCreator  Inputs=7
  Bus Selector2 : BusSelector  OutputSignals=10msTask.BrakeCtrl.BrakingPID_Y,10msTask.BrakeCtrl.BrakingControlActive,INPUTS.DIO_Bus.OperatorEnableSwitch
  Constant10 : Constant  Value=ENUM_XBR_PASS_THROUGH_ACTIVE_T.NOT_ACTIVE
  Constant2 : Constant  Value=-15.687
  Constant4 : Constant  Value=0
  Constant7 : Constant  Value=ENUM_XBR_PASS_THROUGH_ACTIVE_T.ACTIVE
  Constant8 : Constant  Value=ENUM_XBR_PASS_THROUGH_ACTIVE_T.ERROR
  Constant9 : Constant  Value=ENUM_XBR_PASS_THROUGH_ACTIVE_T.NOT_AVAILABLE
  DECEL_GOV_XBR_URGENCY_MPV : Lookup_n-D  NumberOfTableDimensions=1  BreakpointsForDimension1=[-15.687 -2 -1.5 -1.2 -1.1 -1 -0.9 0]  Table=[100 50 20 15 15 15 10 10]  ExtrapMethod=Clip  UseLastTableValue=on  InputSameDT=on
      settings: AttributesFormatString=|
      | X: %<BreakpointsForDimension1>
      | Y: %<Table>
  Divide1 : Product  Inputs=**  InputSameDT=on
  If_Then_Else : EmE_MBD_Blockset/Signal Routing/If_Then_Else
      settings: SourceProductName=PACCAR EmE MBD Blockset
  Multiport Switch : MultiPortSwitch  DataPortOrder=Zero-based contiguous  Inputs=4  DiagnosticForDefault=None  zeroidx=on  InputSameDT=on
  Switch1 : Switch  Criteria=u2 ~= 0
  Terminator1 : Terminator
  XBRControlMode : Constant  Value=ENUM_XBR_CONTROL_MODE_T.ACCEL_CTRL_WITH_MAX_MODE
  XBRControlModeOVR : Constant  Value=ENUM_XBR_CONTROL_MODE_T.ACCEL_CTRL_WITH_MAX_MODE
  XBREnduranceBrakeIntegrationMode : Constant  Value=ENUM_XBR_EBI_MODE_T.EBI_ALLOWED
  XBREnduranceBrakeIntegrationModeOVR : Constant  Value=ENUM_XBR_EBI_MODE_T.EBI_ALLOWED
  XBRExternalAccelDemandOVR : Constant  Value=0
  XBRPassThroughActiveOVR : Constant  Value=ENUM_XBR_PASS_THROUGH_ACTIVE_T.ACTIVE
  XBRPassThroughEnabled : Constant
  XBRPassThroughEnabledOVR : Constant
  XBRPriority : Constant  Value=ENUM_XBR_PRIORITY_T.MEDIUM_PRIORITY
  XBRPriorityOVR : Constant  Value=ENUM_XBR_PRIORITY_T.MEDIUM_PRIORITY
  XBRUrgency : Constant  Value=25
  XBRUrgencyOVR : Constant  Value=25
  XBRValueOverride : Constant  Value=false
  Out : Outport
  wires:
  Constant4/1 -> Switch1/3
  Divide1/1 -> Switch1/1  "XBRExternalAccelDemand"
  Bus Selector2/3 -> Switch1/2  "<OperatorEnableSwitch>"
  Multiport Switch/1 -> Bus Creator1/5  "XBRPassThroughActive"
  DECEL_GOV_XBR_URGENCY_MPV/1 -> Terminator1/1  "XBRUrgency"
  Constant10/1 -> Multiport Switch/2
  Switch1/1 -> Bus Creator1/1, DECEL_GOV_XBR_URGENCY_MPV/1  "XBRExternalAccelDemand"
  Constant2/1 -> Divide1/2
  In/1 -> Bus Selector2/1
  Constant8/1 -> Multiport Switch/4
  Constant9/1 -> Multiport Switch/5
  Constant7/1 -> Multiport Switch/3
  XBREnduranceBrakeIntegrationMode/1 -> Bus Creator1/2  "XBREnduranceBrakeIntegrationMode"
  Bus Selector2/1 -> Divide1/1  "<BrakingPID_Y>"
  Bus Creator1/1 -> If_Then_Else/3
  XBRUrgency/1 -> Bus Creator1/6  "XBRUrgency"
  Bus Selector2/2 -> Multiport Switch/1  "<BrakingControlActive>"
  XBRControlMode/1 -> Bus Creator1/4  "XBRControlMode"
  XBRPriority/1 -> Bus Creator1/3  "XBRPriority"
  XBRPassThroughEnabled/1 -> Bus Creator1/7  "XBRPassThroughEnabled"
  XBRValueOverride/1 -> If_Then_Else/1
  If_Then_Else/1 -> Out/1
  XBRPassThroughActiveOVR/1 -> Bus Creator2/5  "XBRPassThroughActive"
  XBREnduranceBrakeIntegrationModeOVR/1 -> Bus Creator2/2  "XBREnduranceBrakeIntegrationMode"
  XBRExternalAccelDemandOVR/1 -> Bus Creator2/1  "XBRExternalAccelDemand"
  XBRUrgencyOVR/1 -> Bus Creator2/6  "XBRUrgency"
  XBRControlModeOVR/1 -> Bus Creator2/4  "XBRControlMode"
  XBRPriorityOVR/1 -> Bus Creator2/3  "XBRPriority"
  XBRPassThroughEnabledOVR/1 -> Bus Creator2/7  "XBRPassThroughEnabled"
  Bus Creator2/1 -> If_Then_Else/2

== system SUB_ECU_L4_MABX_HW_Interface_PTC_166/CAN_Out_PTC_166/CAN_TX_5000ms/CAN_TX_RQST_13_E4 ==
  RawData : Inport
  OperatorEnable : Inport  Port=2
  Data Type Conversion6 : DataTypeConversion  OutDataTypeStr=boolean  SaturateOnIntegerOverflow=on
  Enable_TX_RequestDiagMsgFromREAX : Constant  Value=boolean(1)
  TX_CAN5 : Subsystem
  wires:
  OperatorEnable/1 -> TX_CAN5/3(OperatorEnable)
  Enable_TX_RequestDiagMsgFromREAX/1 -> Data Type Conversion6/1
  Data Type Conversion6/1 -> TX_CAN5/1(Enable)
  RawData/1 -> TX_CAN5/2(RawData)

== system SUB_ECU_L4_MABX_HW_Interface_PTC_166/CAN_Out_PTC_166/CAN_TX_5000ms/Encode_RQST ==
  PGN : Inport
  AND : PTC_MBDS_LIB/MBDS Standard Library/Basic Operations/Logic and Bit Operations/AND  BitwiseMode=on  Inputs=1  UseBitMask=on  BitMask='000000FF'  OutDataTypeStr=uint8  PTC_MBDS_BlockVersion=5.41  PTC_BlockType=PTC_MBDS_AND
      settings: AttributesFormatString=bitwise  SourceProductName=PACCAR Technical Center MBDS Library
  AND1 : PTC_MBDS_LIB/MBDS Standard Library/Basic Operations/Logic and Bit Operations/AND  BitwiseMode=on  Inputs=1  UseBitMask=on  BitMask='0000FF00'  OutDataTypeStr=uint16  PTC_MBDS_BlockVersion=5.41  PTC_BlockType=PTC_MBDS_AND
      settings: AttributesFormatString=bitwise  SourceProductName=PACCAR Technical Center MBDS Library
  AND2 : PTC_MBDS_LIB/MBDS Standard Library/Basic Operations/Logic and Bit Operations/AND  BitwiseMode=on  Inputs=1  UseBitMask=on  BitMask='00FF0000'  OutDataTypeStr=uint32  PTC_MBDS_BlockVersion=5.41  PTC_BlockType=PTC_MBDS_AND
      settings: AttributesFormatString=bitwise  SourceProductName=PACCAR Technical Center MBDS Library
  Data Type Conversion : DataTypeConversion  OutDataTypeStr=uint32  SaturateOnIntegerOverflow=on
  Data Type Conversion1 : DataTypeConversion  OutDataTypeStr=uint8  SaturateOnIntegerOverflow=on
  Data Type Conversion2 : DataTypeConversion  OutDataTypeStr=uint8  SaturateOnIntegerOverflow=on
  Data Type Conversion3 : DataTypeConversion  OutDataTypeStr=uint8  SaturateOnIntegerOverflow=on
  Mux : Mux  Inputs=3
  "Shift_Arithmetic " : ArithShift  BitShiftNumber=8
  Shift_Arithmetic 1 : ArithShift  BitShiftNumber=16
  Data : Outport
  wires:
  Data Type Conversion3/1 -> Mux/1
  Mux/1 -> Data/1
  Data Type Conversion2/1 -> Mux/3
  Data Type Conversion1/1 -> Mux/2
  Shift_Arithmetic 1/1 -> Data Type Conversion2/1
  AND2/1 -> Shift_Arithmetic 1/1
  "Shift_Arithmetic "/1 -> Data Type Conversion1/1
  AND1/1 -> "Shift_Arithmetic "/1
  AND/1 -> Data Type Conversion3/1
  Data Type Conversion/1 -> AND/1, AND1/1, AND2/1
  PGN/1 -> Data Type Conversion/1

== system SUB_ECU_L4_MABX_HW_Interface_PTC_166/CAN_Out_PTC_166/CAN_TX_5000ms/RQST_13_E4_PGN ==
  Repeating_Sequence_Stair : PTC_MBDS_LIB/Extras/Sources/Repeating_Sequence_Stair  OutValues=uint32([65527, 65226, 65227, 65235, 65242, 65259, 65267, 65260])  OutValues_prev=uint32([65527, 65226, 65227, 65235, 65242, 65259, 65267, 65260])  PTC_MBDS_BlockVersion=5.41  PTC_BlockType=PTC_MBDS_Repeating_Sequence_Stair
      settings: SourceProductName=PACCAR Technical Center MBDS Library
  PGN : Outport
  wires:
  Repeating_Sequence_Stair/1 -> PGN/1
